simulink model "ROPOD_dynamic_model_sim_Wheel_Input"  (R2016b)
settings: Solver=FixedStepAuto  StartTime=0.0  StopTime=timesim(end)  FixedStep=Ts  MaxStep=1e-3  RelTol=1e-3
values from neighbouring files (symbols this model uses):
  ropod_dynmodel_pv = struct2array(ropod_dynmodel_param)    [set_ropod_configparams_sim.m]
(part 4 of 4)

== matlab function ROPOD_dynamic_model_sim_Wheel_Input/Feedback Linearization/m_vector_c ==
  data: ropod_dynmodel_pv input; m output; qin input; dqin input
function m   = m_vector( ropod_dynmodel_pv, qin, dqin)
%ROPOD_JACOBIAN Summary of this function goes here
%   Detailed explanation goes here


r_w     = ropod_dynmodel_pv(1);
s_w     = ropod_dynmodel_pv(2);
d_w     = ropod_dynmodel_pv(3);
l_CW    = ropod_dynmodel_pv(4);

Mr = ropod_dynmodel_pv(5);
Ir = ropod_dynmodel_pv(6);
Mwma = ropod_dynmodel_pv(7);
Iwma = ropod_dynmodel_pv(8);
Mwca = ropod_dynmodel_pv(9);
Iwca = ropod_dynmodel_pv(10);
Mw   = ropod_dynmodel_pv(11);
Iwz  = ropod_dynmodel_pv(12);
Iwp  = ropod_dynmodel_pv(13);

% Map state vector to the corresponfing variables
xc      = qin(1);
yc      = qin(2);
theta   = qin(3);
delta   = qin(4:7);
varphi  = qin(8:15);

% Map state vector to the corresponfing variables
dxc      = dqin(1);
dyc      = dqin(2);
dtheta   = dqin(3);
ddelta   = dqin(4:7);
dvarphi  = dqin(8:15);

delta1 = delta(1);
delta2 = delta(2);
delta3 = delta(3);
delta4 = delta(4);

ddelta1 = ddelta(1);
ddelta2 = ddelta(2);
ddelta3 = ddelta(3);
ddelta4 = ddelta(4);

m = [
                                                                                                                                                                                                                                                                                                                                                                                                                                                                                                                                                                                                                                                                                                                                                                                                                                                                                                                                                                                                                                                                                                                                                                                                                                                                                                                                                                                                                                                                                                                                                                                                                                                                                                                                                                                                                                                                                                                                                                                                                                                                                                                                                                                                                                                                                                                                                                                                                                                                                                                                                                                                                                      dyc*((Iwp*(cos(delta1 + theta) - (d_w*sin(delta1 + theta))/(2*s_w))*(cos(delta1 + theta)*(ddelta1 + dtheta) - (d_w*sin(delta1 + theta)*(ddelta1 + dtheta))/(2*s_w)))/r_w^2 + (Iwp*(cos(delta1 + theta) + (d_w*sin(delta1 + theta))/(2*s_w))*(cos(delta1 + theta)*(ddelta1 + dtheta) + (d_w*sin(delta1 + theta)*(ddelta1 + dtheta))/(2*s_w)))/r_w^2 + (Iwp*(cos(delta2 + theta) - (d_w*sin(delta2 + theta))/(2*s_w))*(cos(delta2 + theta)*(ddelta2 + dtheta) - (d_w*sin(delta2 + theta)*(ddelta2 + dtheta))/(2*s_w)))/r_w^2 + (Iwp*(cos(delta2 + theta) + (d_w*sin(delta2 + theta))/(2*s_w))*(cos(delta2 + theta)*(ddelta2 + dtheta) + (d_w*sin(delta2 + theta)*(ddelta2 + dtheta))/(2*s_w)))/r_w^2 + (Iwp*(cos(delta3 + theta) - (d_w*sin(delta3 + theta))/(2*s_w))*(cos(delta3 + theta)*(ddelta3 + dtheta) - (d_w*sin(delta3 + theta)*(ddelta3 + dtheta))/(2*s_w)))/r_w^2 + (Iwp*(cos(delta3 + theta) + (d_w*sin(delta3 + theta))/(2*s_w))*(cos(delta3 + theta)*(ddelta3 + dtheta) + (d_w*sin(delta3 + theta)*(ddelta3 + dtheta))/(2*s_w)))/r_w^2 + (Iwp*(cos(delta4 + theta) - (d_w*sin(delta4 + theta))/(2*s_w))*(cos(delta4 + theta)*(ddelta4 + dtheta) - (d_w*sin(delta4 + theta)*(ddelta4 + dtheta))/(2*s_w)))/r_w^2 + (Iwp*(cos(delta4 + theta) + (d_w*sin(delta4 + theta))/(2*s_w))*(cos(delta4 + theta)*(ddelta4 + dtheta) + (d_w*sin(delta4 + theta)*(ddelta4 + dtheta))/(2*s_w)))/r_w^2 - (sin(delta1 + theta)*(ddelta1 + dtheta)*(2*Mw*s_w*cos(delta1)*sin(theta) - (sin(delta1 + theta)*(Iwca + Iwma + 2*Iwz + (Mw*d_w^2)/2 + 2*Mw*s_w^2 + (Mwca*s_w^2)/4 + Mwma*s_w^2))/s_w + 2*Mw*s_w*sin(delta1)*cos(theta) + (Mwca*s_w*cos(delta1)*sin(theta))/2 + (Mwca*s_w*sin(delta1)*cos(theta))/2 + Mwma*s_w*cos(delta1)*sin(theta) + Mwma*s_w*sin(delta1)*cos(theta)))/s_w - (sin(delta2 + theta)*(ddelta2 + dtheta)*(2*Mw*s_w*cos(delta2)*sin(theta) - (sin(delta2 + theta)*(Iwca + Iwma + 2*Iwz + (Mw*d_w^2)/2 + 2*Mw*s_w^2 + (Mwca*s_w^2)/4 + Mwma*s_w^2))/s_w + 2*Mw*s_w*sin(delta2)*cos(theta) + (Mwca*s_w*cos(delta2)*sin(theta))/2 + (Mwca*s_w*sin(delta2)*cos(theta))/2 + Mwma*s_w*cos(delta2)*sin(theta) + Mwma*s_w*sin(delta2)*cos(theta)))/s_w - (sin(delta3 + theta)*(ddelta3 + dtheta)*(2*Mw*s_w*cos(delta3)*sin(theta) - (sin(delta3 + theta)*(Iwca + Iwma + 2*Iwz + (Mw*d_w^2)/2 + 2*Mw*s_w^2 + (Mwca*s_w^2)/4 + Mwma*s_w^2))/s_w + 2*Mw*s_w*sin(delta3)*cos(theta) + (Mwca*s_w*cos(delta3)*sin(theta))/2 + (Mwca*s_w*sin(delta3)*cos(theta))/2 + Mwma*s_w*cos(delta3)*sin(theta) + Mwma*s_w*sin(delta3)*cos(theta)))/s_w - (sin(delta4 + theta)*(ddelta4 + dtheta)*(2*Mw*s_w*cos(delta4)*sin(theta) - (sin(delta4 + theta)*(Iwca + Iwma + 2*Iwz + (Mw*d_w^2)/2 + 2*Mw*s_w^2 + (Mwca*s_w^2)/4 + Mwma*s_w^2))/s_w + 2*Mw*s_w*sin(delta4)*cos(theta) + (Mwca*s_w*cos(delta4)*sin(theta))/2 + (Mwca*s_w*sin(delta4)*cos(theta))/2 + Mwma*s_w*cos(delta4)*sin(theta) + Mwma*s_w*sin(delta4)*cos(theta)))/s_w) - dtheta*(((ddelta1*l_CW*sin(delta1) - ddelta1*l_CW*cos(delta1))*(2*Mw*s_w*cos(delta1)*sin(theta) - (sin(delta1 + theta)*(Iwca + Iwma + 2*Iwz + (Mw*d_w^2)/2 + 2*Mw*s_w^2 + (Mwca*s_w^2)/4 + Mwma*s_w^2))/s_w + 2*Mw*s_w*sin(delta1)*cos(theta) + (Mwca*s_w*cos(delta1)*sin(theta))/2 + (Mwca*s_w*sin(delta1)*cos(theta))/2 + Mwma*s_w*cos(delta1)*sin(theta) + Mwma*s_w*sin(delta1)*cos(theta)))/s_w + ((ddelta2*l_CW*sin(delta2) + ddelta2*l_CW*cos(delta2))*(2*Mw*s_w*cos(delta2)*sin(theta) - (sin(delta2 + theta)*(Iwca + Iwma + 2*Iwz + (Mw*d_w^2)/2 + 2*Mw*s_w^2 + (Mwca*s_w^2)/4 + Mwma*s_w^2))/s_w + 2*Mw*s_w*sin(delta2)*cos(theta) + (Mwca*s_w*cos(delta2)*sin(theta))/2 + (Mwca*s_w*sin(delta2)*cos(theta))/2 + Mwma*s_w*cos(delta2)*sin(theta) + Mwma*s_w*sin(delta2)*cos(theta)))/s_w - ((ddelta3*l_CW*sin(delta3) - ddelta3*l_CW*cos(delta3))*(2*Mw*s_w*cos(delta3)*sin(theta) - (sin(delta3 + theta)*(Iwca + Iwma + 2*Iwz + (Mw*d_w^2)/2 + 2*Mw*s_w^2 + (Mwca*s_w^2)/4 + Mwma*s_w^2))/s_w + 2*Mw*s_w*sin(delta3)*cos(theta) + (Mwca*s_w*cos(delta3)*sin(theta))/2 + (Mwca*s_w*sin(delta3)*cos(theta))/2 + Mwma*s_w*cos(delta3)*sin(theta) + Mwma*s_w*sin(delta3)*cos(theta)))/s_w - ((ddelta4*l_CW*sin(delta4) + ddelta4*l_CW*cos(delta4))*(2*Mw*s_w*cos(delta4)*sin(theta) - (sin(delta4 + theta)*(Iwca + Iwma + 2*Iwz + (Mw*d_w^2)/2 + 2*Mw*s_w^2 + (Mwca*s_w^2)/4 + Mwma*s_w^2))/s_w + 2*Mw*s_w*sin(delta4)*cos(theta) + (Mwca*s_w*cos(delta4)*sin(theta))/2 + (Mwca*s_w*sin(delta4)*cos(theta))/2 + Mwma*s_w*cos(delta4)*sin(theta) + Mwma*s_w*sin(delta4)*cos(theta)))/s_w - (Iwp*l_CW*(cos(delta1 + theta) - (d_w*sin(delta1 + theta))/(2*s_w))*(2*ddelta1*s_w*sin(delta1) - d_w*ddelta1*sin(delta1) + d_w*ddelta1*cos(delta1) + 2*ddelta1*s_w*cos(delta1)))/(2*r_w^2*s_w) - (Iwp*l_CW*(cos(delta1 + theta) + (d_w*sin(delta1 + theta))/(2*s_w))*(d_w*ddelta1*sin(delta1) + 2*ddelta1*s_w*sin(delta1) - d_w*ddelta1*cos(delta1) + 2*ddelta1*s_w*cos(delta1)))/(2*r_w^2*s_w) + (Iwp*l_CW*(cos(delta2 + theta) - (d_w*sin(delta2 + theta))/(2*s_w))*(d_w*ddelta2*sin(delta2) + 2*ddelta2*s_w*sin(delta2) + d_w*ddelta2*cos(delta2) - 2*ddelta2*s_w*cos(delta2)))/(2*r_w^2*s_w) - (Iwp*l_CW*(cos(delta2 + theta) + (d_w*sin(delta2 + theta))/(2*s_w))*(d_w*ddelta2*sin(delta2) - 2*ddelta2*s_w*sin(delta2) + d_w*ddelta2*cos(delta2) + 2*ddelta2*s_w*cos(delta2)))/(2*r_w^2*s_w) + (Iwp*l_CW*(cos(delta3 + theta) - (d_w*sin(delta3 + theta))/(2*s_w))*(2*ddelta3*s_w*sin(delta3) - d_w*ddelta3*sin(delta3) + d_w*ddelta3*cos(delta3) + 2*ddelta3*s_w*cos(delta3)))/(2*r_w^2*s_w) + (Iwp*l_CW*(cos(delta3 + theta) + (d_w*sin(delta3 + theta))/(2*s_w))*(d_w*ddelta3*sin(delta3) + 2*ddelta3*s_w*sin(delta3) - d_w*ddelta3*cos(delta3) + 2*ddelta3*s_w*cos(delta3)))/(2*r_w^2*s_w) - (Iwp*l_CW*(cos(delta4 + theta) - (d_w*sin(delta4 + theta))/(2*s_w))*(d_w*ddelta4*sin(delta4) + 2*ddelta4*s_w*sin(delta4) + d_w*ddelta4*cos(delta4) - 2*ddelta4*s_w*cos(delta4)))/(2*r_w^2*s_w) + (Iwp*l_CW*(cos(delta4 + theta) + (d_w*sin(delta4 + theta))/(2*s_w))*(d_w*ddelta4*sin(delta4) - 2*ddelta4*s_w*sin(delta4) + d_w*ddelta4*cos(delta4) + 2*ddelta4*s_w*cos(delta4)))/(2*r_w^2*s_w)) - dxc*((cos(delta1 + theta)*(ddelta1 + dtheta)*(2*Mw*s_w*cos(delta1)*sin(theta) - (sin(delta1 + theta)*(Iwca + Iwma + 2*Iwz + (Mw*d_w^2)/2 + 2*Mw*s_w^2 + (Mwca*s_w^2)/4 + Mwma*s_w^2))/s_w + 2*Mw*s_w*sin(delta1)*cos(theta) + (Mwca*s_w*cos(delta1)*sin(theta))/2 + (Mwca*s_w*sin(delta1)*cos(theta))/2 + Mwma*s_w*cos(delta1)*sin(theta) + Mwma*s_w*sin(delta1)*cos(theta)))/s_w + (cos(delta2 + theta)*(ddelta2 + dtheta)*(2*Mw*s_w*cos(delta2)*sin(theta) - (sin(delta2 + theta)*(Iwca + Iwma + 2*Iwz + (Mw*d_w^2)/2 + 2*Mw*s_w^2 + (Mwca*s_w^2)/4 + Mwma*s_w^2))/s_w + 2*Mw*s_w*sin(delta2)*cos(theta) + (Mwca*s_w*cos(delta2)*sin(theta))/2 + (Mwca*s_w*sin(delta2)*cos(theta))/2 + Mwma*s_w*cos(delta2)*sin(theta) + Mwma*s_w*sin(delta2)*cos(theta)))/s_w + (cos(delta3 + theta)*(ddelta3 + dtheta)*(2*Mw*s_w*cos(delta3)*sin(theta) - (sin(delta3 + theta)*(Iwca + Iwma + 2*Iwz + (Mw*d_w^2)/2 + 2*Mw*s_w^2 + (Mwca*s_w^2)/4 + Mwma*s_w^2))/s_w + 2*Mw*s_w*sin(delta3)*cos(theta) + (Mwca*s_w*cos(delta3)*sin(theta))/2 + (Mwca*s_w*sin(delta3)*cos(theta))/2 + Mwma*s_w*cos(delta3)*sin(theta) + Mwma*s_w*sin(delta3)*cos(theta)))/s_w + (cos(delta4 + theta)*(ddelta4 + dtheta)*(2*Mw*s_w*cos(delta4)*sin(theta) - (sin(delta4 + theta)*(Iwca + Iwma + 2*Iwz + (Mw*d_w^2)/2 + 2*Mw*s_w^2 + (Mwca*s_w^2)/4 + Mwma*s_w^2))/s_w + 2*Mw*s_w*sin(delta4)*cos(theta) + (Mwca*s_w*cos(delta4)*sin(theta))/2 + (Mwca*s_w*sin(delta4)*cos(theta))/2 + Mwma*s_w*cos(delta4)*sin(theta) + Mwma*s_w*sin(delta4)*cos(theta)))/s_w + (Iwp*(cos(delta1 + theta) - (d_w*sin(delta1 + theta))/(2*s_w))*(sin(delta1 + theta)*(ddelta1 + dtheta) + (d_w*cos(delta1 + theta)*(ddelta1 + dtheta))/(2*s_w)))/r_w^2 + (Iwp*(cos(delta1 + theta) + (d_w*sin(delta1 + theta))/(2*s_w))*(sin(delta1 + theta)*(ddelta1 + dtheta) - (d_w*cos(delta1 + theta)*(ddelta1 + dtheta))/(2*s_w)))/r_w^2 + (Iwp*(cos(delta2 + theta) - (d_w*sin(delta2 + theta))/(2*s_w))*(sin(delta2 + theta)*(ddelta2 + dtheta) + (d_w*cos(delta2 + theta)*(ddelta2 + dtheta))/(2*s_w)))/r_w^2 + (Iwp*(cos(delta2 + theta) + (d_w*sin(delta2 + theta))/(2*s_w))*(sin(delta2 + theta)*(ddelta2 + dtheta) - (d_w*cos(delta2 + theta)*(ddelta2 + dtheta))/(2*s_w)))/r_w^2 + (Iwp*(cos(delta3 + theta) - (d_w*sin(delta3 + theta))/(2*s_w))*(sin(delta3 + theta)*(ddelta3 + dtheta) + (d_w*cos(delta3 + theta)*(ddelta3 + dtheta))/(2*s_w)))/r_w^2 + (Iwp*(cos(delta3 + theta) + (d_w*sin(delta3 + theta))/(2*s_w))*(sin(delta3 + theta)*(ddelta3 + dtheta) - (d_w*cos(delta3 + theta)*(ddelta3 + dtheta))/(2*s_w)))/r_w^2 + (Iwp*(cos(delta4 + theta) - (d_w*sin(delta4 + theta))/(2*s_w))*(sin(delta4 + theta)*(ddelta4 + dtheta) + (d_w*cos(delta4 + theta)*(ddelta4 + dtheta))/(2*s_w)))/r_w^2 + (Iwp*(cos(delta4 + theta) + (d_w*sin(delta4 + theta))/(2*s_w))*(sin(delta4 + theta)*(ddelta4 + dtheta) - (d_w*cos(delta4 + theta)*(ddelta4 + dtheta))/(2*s_w)))/r_w^2) + (s_w*(4*Mw + Mwca + 2*Mwma)*(cos(delta1 + theta)*(dtheta*((l_CW*cos(delta1) + l_CW*sin(delta1))/s_w - 1) + (dyc*cos(delta1 + theta))/s_w - (dxc*sin(delta1 + theta))/s_w)^2 + cos(delta2 + theta)*(dtheta*((l_CW*cos(delta2) - l_CW*sin(delta2))/s_w - 1) + (dyc*cos(delta2 + theta))/s_w - (dxc*sin(delta2 + theta))/s_w)^2 + cos(delta3 + theta)*(dtheta*((l_CW*cos(delta3) + l_CW*sin(delta3))/s_w + 1) - (dyc*cos(delta3 + theta))/s_w + (dxc*sin(delta3 + theta))/s_w)^2 + cos(delta4 + theta)*(dtheta*((l_CW*cos(delta4) - l_CW*sin(delta4))/s_w + 1) - (dyc*cos(delta4 + theta))/s_w + (dxc*sin(delta4 + theta))/s_w)^2 + dtheta^2*cos(delta1 + theta) + dtheta^2*cos(delta2 + theta) + dtheta^2*cos(delta3 + theta) + dtheta^2*cos(delta4 + theta) + 2*dtheta*cos(delta1 + theta)*(dtheta*((l_CW*cos(delta1) + l_CW*sin(delta1))/s_w - 1) + (dyc*cos(delta1 + theta))/s_w - (dxc*sin(delta1 + theta))/s_w) + 2*dtheta*cos(delta2 + theta)*(dtheta*((l_CW*cos(delta2) - l_CW*sin(delta2))/s_w - 1) + (dyc*cos(delta2 + theta))/s_w - (dxc*sin(delta2 + theta))/s_w) - 2*dtheta*cos(delta3 + theta)*(dtheta*((l_CW*cos(delta3) + l_CW*sin(delta3))/s_w + 1) - (dyc*cos(delta3 + theta))/s_w + (dxc*sin(delta3 + theta))/s_w) - 2*dtheta*cos(delta4 + theta)*(dtheta*((l_CW*cos(delta4) - l_CW*sin(delta4))/s_w + 1) - (dyc*cos(delta4 + theta))/s_w + (dxc*sin(delta4 + theta))/s_w)))/2 - (2^(1/2)*dtheta^2*l_CW*sin(delta1 + theta)*cos(delta1 + pi/4)*(4*Mw + Mwca + 2*Mwma))/2 + (2^(1/2)*dtheta^2*l_CW*sin(delta3 + theta)*cos(delta3 + pi/4)*(4*Mw + Mwca + 2*Mwma))/2 + (2^(1/2)*dtheta^2*l_CW*sin(delta2 + theta)*sin(delta2 + pi/4)*(4*Mw + Mwca + 2*Mwma))/2 - (2^(1/2)*dtheta^2*l_CW*sin(delta4 + theta)*sin(delta4 + pi/4)*(4*Mw + Mwca + 2*Mwma))/2 ;
                                                                                                                                                                                                                                                                                                                                                                                                                                                                                                                                                                                                                                                                                                                                                                                                                                                                                                                                                                                                                                                                                                                                                                                                                                                                                                                                                                                                                                                                                                                                                                                                                                                                                                                                                                                                                                                                                                                                                                                                                                                                                                                                                                                                                                                                                                                                                                                                                                                                                                                                                                                                                                      dyc*((Iwp*(sin(delta1 + theta) - (d_w*cos(delta1 + theta))/(2*s_w))*(cos(delta1 + theta)*(ddelta1 + dtheta) + (d_w*sin(delta1 + theta)*(ddelta1 + dtheta))/(2*s_w)))/r_w^2 - (sin(delta2 + theta)*(ddelta2 + dtheta)*((cos(delta2 + theta)*(Iwca + Iwma + 2*Iwz + (Mw*d_w^2)/2 + 2*Mw*s_w^2 + (Mwca*s_w^2)/4 + Mwma*s_w^2))/s_w - 2*Mw*s_w*cos(delta2)*cos(theta) - (Mwca*s_w*cos(delta2)*cos(theta))/2 - Mwma*s_w*cos(delta2)*cos(theta) + 2*Mw*s_w*sin(delta2)*sin(theta) + (Mwca*s_w*sin(delta2)*sin(theta))/2 + Mwma*s_w*sin(delta2)*sin(theta)))/s_w - (sin(delta3 + theta)*(ddelta3 + dtheta)*((cos(delta3 + theta)*(Iwca + Iwma + 2*Iwz + (Mw*d_w^2)/2 + 2*Mw*s_w^2 + (Mwca*s_w^2)/4 + Mwma*s_w^2))/s_w - 2*Mw*s_w*cos(delta3)*cos(theta) - (Mwca*s_w*cos(delta3)*cos(theta))/2 - Mwma*s_w*cos(delta3)*cos(theta) + 2*Mw*s_w*sin(delta3)*sin(theta) + (Mwca*s_w*sin(delta3)*sin(theta))/2 + Mwma*s_w*sin(delta3)*sin(theta)))/s_w - (sin(delta4 + theta)*(ddelta4 + dtheta)*((cos(delta4 + theta)*(Iwca + Iwma + 2*Iwz + (Mw*d_w^2)/2 + 2*Mw*s_w^2 + (Mwca*s_w^2)/4 + Mwma*s_w^2))/s_w - 2*Mw*s_w*cos(delta4)*cos(theta) - (Mwca*s_w*cos(delta4)*cos(theta))/2 - Mwma*s_w*cos(delta4)*cos(theta) + 2*Mw*s_w*sin(delta4)*sin(theta) + (Mwca*s_w*sin(delta4)*sin(theta))/2 + Mwma*s_w*sin(delta4)*sin(theta)))/s_w - (sin(delta1 + theta)*(ddelta1 + dtheta)*((cos(delta1 + theta)*(Iwca + Iwma + 2*Iwz + (Mw*d_w^2)/2 + 2*Mw*s_w^2 + (Mwca*s_w^2)/4 + Mwma*s_w^2))/s_w - 2*Mw*s_w*cos(delta1)*cos(theta) - (Mwca*s_w*cos(delta1)*cos(theta))/2 - Mwma*s_w*cos(delta1)*cos(theta) + 2*Mw*s_w*sin(delta1)*sin(theta) + (Mwca*s_w*sin(delta1)*sin(theta))/2 + Mwma*s_w*sin(delta1)*sin(theta)))/s_w + (Iwp*(sin(delta1 + theta) + (d_w*cos(delta1 + theta))/(2*s_w))*(cos(delta1 + theta)*(ddelta1 + dtheta) - (d_w*sin(delta1 + theta)*(ddelta1 + dtheta))/(2*s_w)))/r_w^2 + (Iwp*(sin(delta2 + theta) - (d_w*cos(delta2 + theta))/(2*s_w))*(cos(delta2 + theta)*(ddelta2 + dtheta) + (d_w*sin(delta2 + theta)*(ddelta2 + dtheta))/(2*s_w)))/r_w^2 + (Iwp*(sin(delta2 + theta) + (d_w*cos(delta2 + theta))/(2*s_w))*(cos(delta2 + theta)*(ddelta2 + dtheta) - (d_w*sin(delta2 + theta)*(ddelta2 + dtheta))/(2*s_w)))/r_w^2 + (Iwp*(sin(delta3 + theta) - (d_w*cos(delta3 + theta))/(2*s_w))*(cos(delta3 + theta)*(ddelta3 + dtheta) + (d_w*sin(delta3 + theta)*(ddelta3 + dtheta))/(2*s_w)))/r_w^2 + (Iwp*(sin(delta3 + theta) + (d_w*cos(delta3 + theta))/(2*s_w))*(cos(delta3 + theta)*(ddelta3 + dtheta) - (d_w*sin(delta3 + theta)*(ddelta3 + dtheta))/(2*s_w)))/r_w^2 + (Iwp*(sin(delta4 + theta) - (d_w*cos(delta4 + theta))/(2*s_w))*(cos(delta4 + theta)*(ddelta4 + dtheta) + (d_w*sin(delta4 + theta)*(ddelta4 + dtheta))/(2*s_w)))/r_w^2 + (Iwp*(sin(delta4 + theta) + (d_w*cos(delta4 + theta))/(2*s_w))*(cos(delta4 + theta)*(ddelta4 + dtheta) - (d_w*sin(delta4 + theta)*(ddelta4 + dtheta))/(2*s_w)))/r_w^2) - dxc*((cos(delta1 + theta)*(ddelta1 + dtheta)*((cos(delta1 + theta)*(Iwca + Iwma + 2*Iwz + (Mw*d_w^2)/2 + 2*Mw*s_w^2 + (Mwca*s_w^2)/4 + Mwma*s_w^2))/s_w - 2*Mw*s_w*cos(delta1)*cos(theta) - (Mwca*s_w*cos(delta1)*cos(theta))/2 - Mwma*s_w*cos(delta1)*cos(theta) + 2*Mw*s_w*sin(delta1)*sin(theta) + (Mwca*s_w*sin(delta1)*sin(theta))/2 + Mwma*s_w*sin(delta1)*sin(theta)))/s_w + (cos(delta2 + theta)*(ddelta2 + dtheta)*((cos(delta2 + theta)*(Iwca + Iwma + 2*Iwz + (Mw*d_w^2)/2 + 2*Mw*s_w^2 + (Mwca*s_w^2)/4 + Mwma*s_w^2))/s_w - 2*Mw*s_w*cos(delta2)*cos(theta) - (Mwca*s_w*cos(delta2)*cos(theta))/2 - Mwma*s_w*cos(delta2)*cos(theta) + 2*Mw*s_w*sin(delta2)*sin(theta) + (Mwca*s_w*sin(delta2)*sin(theta))/2 + Mwma*s_w*sin(delta2)*sin(theta)))/s_w + (cos(delta3 + theta)*(ddelta3 + dtheta)*((cos(delta3 + theta)*(Iwca + Iwma + 2*Iwz + (Mw*d_w^2)/2 + 2*Mw*s_w^2 + (Mwca*s_w^2)/4 + Mwma*s_w^2))/s_w - 2*Mw*s_w*cos(delta3)*cos(theta) - (Mwca*s_w*cos(delta3)*cos(theta))/2 - Mwma*s_w*cos(delta3)*cos(theta) + 2*Mw*s_w*sin(delta3)*sin(theta) + (Mwca*s_w*sin(delta3)*sin(theta))/2 + Mwma*s_w*sin(delta3)*sin(theta)))/s_w + (cos(delta4 + theta)*(ddelta4 + dtheta)*((cos(delta4 + theta)*(Iwca + Iwma + 2*Iwz + (Mw*d_w^2)/2 + 2*Mw*s_w^2 + (Mwca*s_w^2)/4 + Mwma*s_w^2))/s_w - 2*Mw*s_w*cos(delta4)*cos(theta) - (Mwca*s_w*cos(delta4)*cos(theta))/2 - Mwma*s_w*cos(delta4)*cos(theta) + 2*Mw*s_w*sin(delta4)*sin(theta) + (Mwca*s_w*sin(delta4)*sin(theta))/2 + Mwma*s_w*sin(delta4)*sin(theta)))/s_w + (Iwp*(sin(delta1 + theta) - (d_w*cos(delta1 + theta))/(2*s_w))*(sin(delta1 + theta)*(ddelta1 + dtheta) - (d_w*cos(delta1 + theta)*(ddelta1 + dtheta))/(2*s_w)))/r_w^2 + (Iwp*(sin(delta1 + theta) + (d_w*cos(delta1 + theta))/(2*s_w))*(sin(delta1 + theta)*(ddelta1 + dtheta) + (d_w*cos(delta1 + theta)*(ddelta1 + dtheta))/(2*s_w)))/r_w^2 + (Iwp*(sin(delta2 + theta) - (d_w*cos(delta2 + theta))/(2*s_w))*(sin(delta2 + theta)*(ddelta2 + dtheta) - (d_w*cos(delta2 + theta)*(ddelta2 + dtheta))/(2*s_w)))/r_w^2 + (Iwp*(sin(delta2 + theta) + (d_w*cos(delta2 + theta))/(2*s_w))*(sin(delta2 + theta)*(ddelta2 + dtheta) + (d_w*cos(delta2 + theta)*(ddelta2 + dtheta))/(2*s_w)))/r_w^2 + (Iwp*(sin(delta3 + theta) - (d_w*cos(delta3 + theta))/(2*s_w))*(sin(delta3 + theta)*(ddelta3 + dtheta) - (d_w*cos(delta3 + theta)*(ddelta3 + dtheta))/(2*s_w)))/r_w^2 + (Iwp*(sin(delta3 + theta) + (d_w*cos(delta3 + theta))/(2*s_w))*(sin(delta3 + theta)*(ddelta3 + dtheta) + (d_w*cos(delta3 + theta)*(ddelta3 + dtheta))/(2*s_w)))/r_w^2 + (Iwp*(sin(delta4 + theta) - (d_w*cos(delta4 + theta))/(2*s_w))*(sin(delta4 + theta)*(ddelta4 + dtheta) - (d_w*cos(delta4 + theta)*(ddelta4 + dtheta))/(2*s_w)))/r_w^2 + (Iwp*(sin(delta4 + theta) + (d_w*cos(delta4 + theta))/(2*s_w))*(sin(delta4 + theta)*(ddelta4 + dtheta) + (d_w*cos(delta4 + theta)*(ddelta4 + dtheta))/(2*s_w)))/r_w^2) - dtheta*(((ddelta1*l_CW*sin(delta1) - ddelta1*l_CW*cos(delta1))*((cos(delta1 + theta)*(Iwca + Iwma + 2*Iwz + (Mw*d_w^2)/2 + 2*Mw*s_w^2 + (Mwca*s_w^2)/4 + Mwma*s_w^2))/s_w - 2*Mw*s_w*cos(delta1)*cos(theta) - (Mwca*s_w*cos(delta1)*cos(theta))/2 - Mwma*s_w*cos(delta1)*cos(theta) + 2*Mw*s_w*sin(delta1)*sin(theta) + (Mwca*s_w*sin(delta1)*sin(theta))/2 + Mwma*s_w*sin(delta1)*sin(theta)))/s_w + ((ddelta2*l_CW*sin(delta2) + ddelta2*l_CW*cos(delta2))*((cos(delta2 + theta)*(Iwca + Iwma + 2*Iwz + (Mw*d_w^2)/2 + 2*Mw*s_w^2 + (Mwca*s_w^2)/4 + Mwma*s_w^2))/s_w - 2*Mw*s_w*cos(delta2)*cos(theta) - (Mwca*s_w*cos(delta2)*cos(theta))/2 - Mwma*s_w*cos(delta2)*cos(theta) + 2*Mw*s_w*sin(delta2)*sin(theta) + (Mwca*s_w*sin(delta2)*sin(theta))/2 + Mwma*s_w*sin(delta2)*sin(theta)))/s_w - ((ddelta3*l_CW*sin(delta3) - ddelta3*l_CW*cos(delta3))*((cos(delta3 + theta)*(Iwca + Iwma + 2*Iwz + (Mw*d_w^2)/2 + 2*Mw*s_w^2 + (Mwca*s_w^2)/4 + Mwma*s_w^2))/s_w - 2*Mw*s_w*cos(delta3)*cos(theta) - (Mwca*s_w*cos(delta3)*cos(theta))/2 - Mwma*s_w*cos(delta3)*cos(theta) + 2*Mw*s_w*sin(delta3)*sin(theta) + (Mwca*s_w*sin(delta3)*sin(theta))/2 + Mwma*s_w*sin(delta3)*sin(theta)))/s_w - ((ddelta4*l_CW*sin(delta4) + ddelta4*l_CW*cos(delta4))*((cos(delta4 + theta)*(Iwca + Iwma + 2*Iwz + (Mw*d_w^2)/2 + 2*Mw*s_w^2 + (Mwca*s_w^2)/4 + Mwma*s_w^2))/s_w - 2*Mw*s_w*cos(delta4)*cos(theta) - (Mwca*s_w*cos(delta4)*cos(theta))/2 - Mwma*s_w*cos(delta4)*cos(theta) + 2*Mw*s_w*sin(delta4)*sin(theta) + (Mwca*s_w*sin(delta4)*sin(theta))/2 + Mwma*s_w*sin(delta4)*sin(theta)))/s_w - (Iwp*l_CW*(sin(delta1 + theta) - (d_w*cos(delta1 + theta))/(2*s_w))*(d_w*ddelta1*sin(delta1) + 2*ddelta1*s_w*sin(delta1) - d_w*ddelta1*cos(delta1) + 2*ddelta1*s_w*cos(delta1)))/(2*r_w^2*s_w) - (Iwp*l_CW*(sin(delta1 + theta) + (d_w*cos(delta1 + theta))/(2*s_w))*(2*ddelta1*s_w*sin(delta1) - d_w*ddelta1*sin(delta1) + d_w*ddelta1*cos(delta1) + 2*ddelta1*s_w*cos(delta1)))/(2*r_w^2*s_w) - (Iwp*l_CW*(sin(delta2 + theta) - (d_w*cos(delta2 + theta))/(2*s_w))*(d_w*ddelta2*sin(delta2) - 2*ddelta2*s_w*sin(delta2) + d_w*ddelta2*cos(delta2) + 2*ddelta2*s_w*cos(delta2)))/(2*r_w^2*s_w) + (Iwp*l_CW*(sin(delta2 + theta) + (d_w*cos(delta2 + theta))/(2*s_w))*(d_w*ddelta2*sin(delta2) + 2*ddelta2*s_w*sin(delta2) + d_w*ddelta2*cos(delta2) - 2*ddelta2*s_w*cos(delta2)))/(2*r_w^2*s_w) + (Iwp*l_CW*(sin(delta3 + theta) - (d_w*cos(delta3 + theta))/(2*s_w))*(d_w*ddelta3*sin(delta3) + 2*ddelta3*s_w*sin(delta3) - d_w*ddelta3*cos(delta3) + 2*ddelta3*s_w*cos(delta3)))/(2*r_w^2*s_w) + (Iwp*l_CW*(sin(delta3 + theta) + (d_w*cos(delta3 + theta))/(2*s_w))*(2*ddelta3*s_w*sin(delta3) - d_w*ddelta3*sin(delta3) + d_w*ddelta3*cos(delta3) + 2*ddelta3*s_w*cos(delta3)))/(2*r_w^2*s_w) + (Iwp*l_CW*(sin(delta4 + theta) - (d_w*cos(delta4 + theta))/(2*s_w))*(d_w*ddelta4*sin(delta4) - 2*ddelta4*s_w*sin(delta4) + d_w*ddelta4*cos(delta4) + 2*ddelta4*s_w*cos(delta4)))/(2*r_w^2*s_w) - (Iwp*l_CW*(sin(delta4 + theta) + (d_w*cos(delta4 + theta))/(2*s_w))*(d_w*ddelta4*sin(delta4) + 2*ddelta4*s_w*sin(delta4) + d_w*ddelta4*cos(delta4) - 2*ddelta4*s_w*cos(delta4)))/(2*r_w^2*s_w)) + (s_w*(4*Mw + Mwca + 2*Mwma)*(sin(delta1 + theta)*(dtheta*((l_CW*cos(delta1) + l_CW*sin(delta1))/s_w - 1) + (dyc*cos(delta1 + theta))/s_w - (dxc*sin(delta1 + theta))/s_w)^2 + sin(delta2 + theta)*(dtheta*((l_CW*cos(delta2) - l_CW*sin(delta2))/s_w - 1) + (dyc*cos(delta2 + theta))/s_w - (dxc*sin(delta2 + theta))/s_w)^2 + sin(delta3 + theta)*(dtheta*((l_CW*cos(delta3) + l_CW*sin(delta3))/s_w + 1) - (dyc*cos(delta3 + theta))/s_w + (dxc*sin(delta3 + theta))/s_w)^2 + sin(delta4 + theta)*(dtheta*((l_CW*cos(delta4) - l_CW*sin(delta4))/s_w + 1) - (dyc*cos(delta4 + theta))/s_w + (dxc*sin(delta4 + theta))/s_w)^2 + dtheta^2*sin(delta1 + theta) + dtheta^2*sin(delta2 + theta) + dtheta^2*sin(delta3 + theta) + dtheta^2*sin(delta4 + theta) + 2*dtheta*sin(delta1 + theta)*(dtheta*((l_CW*cos(delta1) + l_CW*sin(delta1))/s_w - 1) + (dyc*cos(delta1 + theta))/s_w - (dxc*sin(delta1 + theta))/s_w) + 2*dtheta*sin(delta2 + theta)*(dtheta*((l_CW*cos(delta2) - l_CW*sin(delta2))/s_w - 1) + (dyc*cos(delta2 + theta))/s_w - (dxc*sin(delta2 + theta))/s_w) - 2*dtheta*sin(delta3 + theta)*(dtheta*((l_CW*cos(delta3) + l_CW*sin(delta3))/s_w + 1) - (dyc*cos(delta3 + theta))/s_w + (dxc*sin(delta3 + theta))/s_w) - 2*dtheta*sin(delta4 + theta)*(dtheta*((l_CW*cos(delta4) - l_CW*sin(delta4))/s_w + 1) - (dyc*cos(delta4 + theta))/s_w + (dxc*sin(delta4 + theta))/s_w)))/2 + (2^(1/2)*dtheta^2*l_CW*cos(delta1 + theta)*cos(delta1 + pi/4)*(4*Mw + Mwca + 2*Mwma))/2 - (2^(1/2)*dtheta^2*l_CW*cos(delta3 + theta)*cos(delta3 + pi/4)*(4*Mw + Mwca + 2*Mwma))/2 - (2^(1/2)*dtheta^2*l_CW*cos(delta2 + theta)*sin(delta2 + pi/4)*(4*Mw + Mwca + 2*Mwma))/2 + (2^(1/2)*dtheta^2*l_CW*cos(delta4 + theta)*sin(delta4 + pi/4)*(4*Mw + Mwca + 2*Mwma))/2 ;
 (l_CW*s_w*(4*Mw + Mwca + 2*Mwma)*(cos(delta2)*(dtheta*((l_CW*cos(delta2) - l_CW*sin(delta2))/s_w - 1) + (dyc*cos(delta2 + theta))/s_w - (dxc*sin(delta2 + theta))/s_w)^2 - cos(delta1)*(dtheta*((l_CW*cos(delta1) + l_CW*sin(delta1))/s_w - 1) + (dyc*cos(delta1 + theta))/s_w - (dxc*sin(delta1 + theta))/s_w)^2 + cos(delta3)*(dtheta*((l_CW*cos(delta3) + l_CW*sin(delta3))/s_w + 1) - (dyc*cos(delta3 + theta))/s_w + (dxc*sin(delta3 + theta))/s_w)^2 - cos(delta4)*(dtheta*((l_CW*cos(delta4) - l_CW*sin(delta4))/s_w + 1) - (dyc*cos(delta4 + theta))/s_w + (dxc*sin(delta4 + theta))/s_w)^2 + sin(delta1)*(dtheta*((l_CW*cos(delta1) + l_CW*sin(delta1))/s_w - 1) + (dyc*cos(delta1 + theta))/s_w - (dxc*sin(delta1 + theta))/s_w)^2 + sin(delta2)*(dtheta*((l_CW*cos(delta2) - l_CW*sin(delta2))/s_w - 1) + (dyc*cos(delta2 + theta))/s_w - (dxc*sin(delta2 + theta))/s_w)^2 - sin(delta3)*(dtheta*((l_CW*cos(delta3) + l_CW*sin(delta3))/s_w + 1) - (dyc*cos(delta3 + theta))/s_w + (dxc*sin(delta3 + theta))/s_w)^2 - sin(delta4)*(dtheta*((l_CW*cos(delta4) - l_CW*sin(delta4))/s_w + 1) - (dyc*cos(delta4 + theta))/s_w + (dxc*sin(delta4 + theta))/s_w)^2 - 2*dtheta*cos(delta1)*(dtheta*((l_CW*cos(delta1) + l_CW*sin(delta1))/s_w - 1) + (dyc*cos(delta1 + theta))/s_w - (dxc*sin(delta1 + theta))/s_w) + 2*dtheta*cos(delta2)*(dtheta*((l_CW*cos(delta2) - l_CW*sin(delta2))/s_w - 1) + (dyc*cos(delta2 + theta))/s_w - (dxc*sin(delta2 + theta))/s_w) - 2*dtheta*cos(delta3)*(dtheta*((l_CW*cos(delta3) + l_CW*sin(delta3))/s_w + 1) - (dyc*cos(delta3 + theta))/s_w + (dxc*sin(delta3 + theta))/s_w) + 2*dtheta*cos(delta4)*(dtheta*((l_CW*cos(delta4) - l_CW*sin(delta4))/s_w + 1) - (dyc*cos(delta4 + theta))/s_w + (dxc*sin(delta4 + theta))/s_w) + 2*dtheta*sin(delta1)*(dtheta*((l_CW*cos(delta1) + l_CW*sin(delta1))/s_w - 1) + (dyc*cos(delta1 + theta))/s_w - (dxc*sin(delta1 + theta))/s_w) + 2*dtheta*sin(delta2)*(dtheta*((l_CW*cos(delta2) - l_CW*sin(delta2))/s_w - 1) + (dyc*cos(delta2 + theta))/s_w - (dxc*sin(delta2 + theta))/s_w) + 2*dtheta*sin(delta3)*(dtheta*((l_CW*cos(delta3) + l_CW*sin(delta3))/s_w + 1) - (dyc*cos(delta3 + theta))/s_w + (dxc*sin(delta3 + theta))/s_w) + 2*dtheta*sin(delta4)*(dtheta*((l_CW*cos(delta4) - l_CW*sin(delta4))/s_w + 1) - (dyc*cos(delta4 + theta))/s_w + (dxc*sin(delta4 + theta))/s_w)))/2 - dxc*((cos(delta1 + theta)*(ddelta1 + dtheta)*(Iwca + Iwma + 2*Iwz + ((l_CW*cos(delta1) + l_CW*sin(delta1))/s_w - 1)*(Iwca + Iwma + 2*Iwz + (Mw*d_w^2)/2 + 2*Mw*s_w^2 + (Mwca*s_w^2)/4 + Mwma*s_w^2) + (Mw*d_w^2)/2 + 2*Mw*s_w^2 + (Mwca*s_w^2)/4 + Mwma*s_w^2 - 2*Mw*l_CW*s_w*cos(delta1) - (Mwca*l_CW*s_w*cos(delta1))/2 - Mwma*l_CW*s_w*cos(delta1) - 2*Mw*l_CW*s_w*sin(delta1) - (Mwca*l_CW*s_w*sin(delta1))/2 - Mwma*l_CW*s_w*sin(delta1)))/s_w + (cos(delta2 + theta)*(ddelta2 + dtheta)*(Iwca + Iwma + 2*Iwz + ((l_CW*cos(delta2) - l_CW*sin(delta2))/s_w - 1)*(Iwca + Iwma + 2*Iwz + (Mw*d_w^2)/2 + 2*Mw*s_w^2 + (Mwca*s_w^2)/4 + Mwma*s_w^2) + (Mw*d_w^2)/2 + 2*Mw*s_w^2 + (Mwca*s_w^2)/4 + Mwma*s_w^2 - 2*Mw*l_CW*s_w*cos(delta2) - (Mwca*l_CW*s_w*cos(delta2))/2 - Mwma*l_CW*s_w*cos(delta2) + 2*Mw*l_CW*s_w*sin(delta2) + (Mwca*l_CW*s_w*sin(delta2))/2 + Mwma*l_CW*s_w*sin(delta2)))/s_w + (cos(delta3 + theta)*(ddelta3 + dtheta)*(Iwca + Iwma + 2*Iwz - ((l_CW*cos(delta3) + l_CW*sin(delta3))/s_w + 1)*(Iwca + Iwma + 2*Iwz + (Mw*d_w^2)/2 + 2*Mw*s_w^2 + (Mwca*s_w^2)/4 + Mwma*s_w^2) + (Mw*d_w^2)/2 + 2*Mw*s_w^2 + (Mwca*s_w^2)/4 + Mwma*s_w^2 + 2*Mw*l_CW*s_w*cos(delta3) + (Mwca*l_CW*s_w*cos(delta3))/2 + Mwma*l_CW*s_w*cos(delta3) + 2*Mw*l_CW*s_w*sin(delta3) + (Mwca*l_CW*s_w*sin(delta3))/2 + Mwma*l_CW*s_w*sin(delta3)))/s_w + (cos(delta4 + theta)*(ddelta4 + dtheta)*(Iwca + Iwma + 2*Iwz - ((l_CW*cos(delta4) - l_CW*sin(delta4))/s_w + 1)*(Iwca + Iwma + 2*Iwz + (Mw*d_w^2)/2 + 2*Mw*s_w^2 + (Mwca*s_w^2)/4 + Mwma*s_w^2) + (Mw*d_w^2)/2 + 2*Mw*s_w^2 + (Mwca*s_w^2)/4 + Mwma*s_w^2 + 2*Mw*l_CW*s_w*cos(delta4) + (Mwca*l_CW*s_w*cos(delta4))/2 + Mwma*l_CW*s_w*cos(delta4) - 2*Mw*l_CW*s_w*sin(delta4) - (Mwca*l_CW*s_w*sin(delta4))/2 - Mwma*l_CW*s_w*sin(delta4)))/s_w - (Iwp*l_CW*(sin(delta1 + theta)*(ddelta1 + dtheta) - (d_w*cos(delta1 + theta)*(ddelta1 + dtheta))/(2*s_w))*(d_w*cos(delta1) + 2*s_w*cos(delta1) + d_w*sin(delta1) - 2*s_w*sin(delta1)))/(2*r_w^2*s_w) + (Iwp*l_CW*(sin(delta1 + theta)*(ddelta1 + dtheta) + (d_w*cos(delta1 + theta)*(ddelta1 + dtheta))/(2*s_w))*(d_w*cos(delta1) - 2*s_w*cos(delta1) + d_w*sin(delta1) + 2*s_w*sin(delta1)))/(2*r_w^2*s_w) + (Iwp*l_CW*(sin(delta2 + theta)*(ddelta2 + dtheta) - (d_w*cos(delta2 + theta)*(ddelta2 + dtheta))/(2*s_w))*(2*s_w*cos(delta2) - d_w*cos(delta2) + d_w*sin(delta2) + 2*s_w*sin(delta2)))/(2*r_w^2*s_w) + (Iwp*l_CW*(sin(delta2 + theta)*(ddelta2 + dtheta) + (d_w*cos(delta2 + theta)*(ddelta2 + dtheta))/(2*s_w))*(d_w*cos(delta2) + 2*s_w*cos(delta2) - d_w*sin(delta2) + 2*s_w*sin(delta2)))/(2*r_w^2*s_w) + (Iwp*l_CW*(sin(delta3 + theta)*(ddelta3 + dtheta) - (d_w*cos(delta3 + theta)*(ddelta3 + dtheta))/(2*s_w))*(d_w*cos(delta3) + 2*s_w*cos(delta3) + d_w*sin(delta3) - 2*s_w*sin(delta3)))/(2*r_w^2*s_w) - (Iwp*l_CW*(sin(delta3 + theta)*(ddelta3 + dtheta) + (d_w*cos(delta3 + theta)*(ddelta3 + dtheta))/(2*s_w))*(d_w*cos(delta3) - 2*s_w*cos(delta3) + d_w*sin(delta3) + 2*s_w*sin(delta3)))/(2*r_w^2*s_w) - (Iwp*l_CW*(sin(delta4 + theta)*(ddelta4 + dtheta) - (d_w*cos(delta4 + theta)*(ddelta4 + dtheta))/(2*s_w))*(2*s_w*cos(delta4) - d_w*cos(delta4) + d_w*sin(delta4) + 2*s_w*sin(delta4)))/(2*r_w^2*s_w) - (Iwp*l_CW*(sin(delta4 + theta)*(ddelta4 + dtheta) + (d_w*cos(delta4 + theta)*(ddelta4 + dtheta))/(2*s_w))*(d_w*cos(delta4) + 2*s_w*cos(delta4) - d_w*sin(delta4) + 2*s_w*sin(delta4)))/(2*r_w^2*s_w)) - dyc*((sin(delta1 + theta)*(ddelta1 + dtheta)*(Iwca + Iwma + 2*Iwz + ((l_CW*cos(delta1) + l_CW*sin(delta1))/s_w - 1)*(Iwca + Iwma + 2*Iwz + (Mw*d_w^2)/2 + 2*Mw*s_w^2 + (Mwca*s_w^2)/4 + Mwma*s_w^2) + (Mw*d_w^2)/2 + 2*Mw*s_w^2 + (Mwca*s_w^2)/4 + Mwma*s_w^2 - 2*Mw*l_CW*s_w*cos(delta1) - (Mwca*l_CW*s_w*cos(delta1))/2 - Mwma*l_CW*s_w*cos(delta1) - 2*Mw*l_CW*s_w*sin(delta1) - (Mwca*l_CW*s_w*sin(delta1))/2 - Mwma*l_CW*s_w*sin(delta1)))/s_w + (sin(delta2 + theta)*(ddelta2 + dtheta)*(Iwca + Iwma + 2*Iwz + ((l_CW*cos(delta2) - l_CW*sin(delta2))/s_w - 1)*(Iwca + Iwma + 2*Iwz + (Mw*d_w^2)/2 + 2*Mw*s_w^2 + (Mwca*s_w^2)/4 + Mwma*s_w^2) + (Mw*d_w^2)/2 + 2*Mw*s_w^2 + (Mwca*s_w^2)/4 + Mwma*s_w^2 - 2*Mw*l_CW*s_w*cos(delta2) - (Mwca*l_CW*s_w*cos(delta2))/2 - Mwma*l_CW*s_w*cos(delta2) + 2*Mw*l_CW*s_w*sin(delta2) + (Mwca*l_CW*s_w*sin(delta2))/2 + Mwma*l_CW*s_w*sin(delta2)))/s_w + (sin(delta3 + theta)*(ddelta3 + dtheta)*(Iwca + Iwma + 2*Iwz - ((l_CW*cos(delta3) + l_CW*sin(delta3))/s_w + 1)*(Iwca + Iwma + 2*Iwz + (Mw*d_w^2)/2 + 2*Mw*s_w^2 + (Mwca*s_w^2)/4 + Mwma*s_w^2) + (Mw*d_w^2)/2 + 2*Mw*s_w^2 + (Mwca*s_w^2)/4 + Mwma*s_w^2 + 2*Mw*l_CW*s_w*cos(delta3) + (Mwca*l_CW*s_w*cos(delta3))/2 + Mwma*l_CW*s_w*cos(delta3) + 2*Mw*l_CW*s_w*sin(delta3) + (Mwca*l_CW*s_w*sin(delta3))/2 + Mwma*l_CW*s_w*sin(delta3)))/s_w + (sin(delta4 + theta)*(ddelta4 + dtheta)*(Iwca + Iwma + 2*Iwz - ((l_CW*cos(delta4) - l_CW*sin(delta4))/s_w + 1)*(Iwca + Iwma + 2*Iwz + (Mw*d_w^2)/2 + 2*Mw*s_w^2 + (Mwca*s_w^2)/4 + Mwma*s_w^2) + (Mw*d_w^2)/2 + 2*Mw*s_w^2 + (Mwca*s_w^2)/4 + Mwma*s_w^2 + 2*Mw*l_CW*s_w*cos(delta4) + (Mwca*l_CW*s_w*cos(delta4))/2 + Mwma*l_CW*s_w*cos(delta4) - 2*Mw*l_CW*s_w*sin(delta4) - (Mwca*l_CW*s_w*sin(delta4))/2 - Mwma*l_CW*s_w*sin(delta4)))/s_w - (Iwp*l_CW*(cos(delta1 + theta)*(ddelta1 + dtheta) - (d_w*sin(delta1 + theta)*(ddelta1 + dtheta))/(2*s_w))*(d_w*cos(delta1) - 2*s_w*cos(delta1) + d_w*sin(delta1) + 2*s_w*sin(delta1)))/(2*r_w^2*s_w) + (Iwp*l_CW*(cos(delta1 + theta)*(ddelta1 + dtheta) + (d_w*sin(delta1 + theta)*(ddelta1 + dtheta))/(2*s_w))*(d_w*cos(delta1) + 2*s_w*cos(delta1) + d_w*sin(delta1) - 2*s_w*sin(delta1)))/(2*r_w^2*s_w) - (Iwp*l_CW*(cos(delta2 + theta)*(ddelta2 + dtheta) - (d_w*sin(delta2 + theta)*(ddelta2 + dtheta))/(2*s_w))*(d_w*cos(delta2) + 2*s_w*cos(delta2) - d_w*sin(delta2) + 2*s_w*sin(delta2)))/(2*r_w^2*s_w) - (Iwp*l_CW*(cos(delta2 + theta)*(ddelta2 + dtheta) + (d_w*sin(delta2 + theta)*(ddelta2 + dtheta))/(2*s_w))*(2*s_w*cos(delta2) - d_w*cos(delta2) + d_w*sin(delta2) + 2*s_w*sin(delta2)))/(2*r_w^2*s_w) + (Iwp*l_CW*(cos(delta3 + theta)*(ddelta3 + dtheta) - (d_w*sin(delta3 + theta)*(ddelta3 + dtheta))/(2*s_w))*(d_w*cos(delta3) - 2*s_w*cos(delta3) + d_w*sin(delta3) + 2*s_w*sin(delta3)))/(2*r_w^2*s_w) - (Iwp*l_CW*(cos(delta3 + theta)*(ddelta3 + dtheta) + (d_w*sin(delta3 + theta)*(ddelta3 + dtheta))/(2*s_w))*(d_w*cos(delta3) + 2*s_w*cos(delta3) + d_w*sin(delta3) - 2*s_w*sin(delta3)))/(2*r_w^2*s_w) + (Iwp*l_CW*(cos(delta4 + theta)*(ddelta4 + dtheta) - (d_w*sin(delta4 + theta)*(ddelta4 + dtheta))/(2*s_w))*(d_w*cos(delta4) + 2*s_w*cos(delta4) - d_w*sin(delta4) + 2*s_w*sin(delta4)))/(2*r_w^2*s_w) + (Iwp*l_CW*(cos(delta4 + theta)*(ddelta4 + dtheta) + (d_w*sin(delta4 + theta)*(ddelta4 + dtheta))/(2*s_w))*(2*s_w*cos(delta4) - d_w*cos(delta4) + d_w*sin(delta4) + 2*s_w*sin(delta4)))/(2*r_w^2*s_w)) - dtheta*(((ddelta1*l_CW*sin(delta1) - ddelta1*l_CW*cos(delta1))*(Iwca + Iwma + 2*Iwz + ((l_CW*cos(delta1) + l_CW*sin(delta1))/s_w - 1)*(Iwca + Iwma + 2*Iwz + (Mw*d_w^2)/2 + 2*Mw*s_w^2 + (Mwca*s_w^2)/4 + Mwma*s_w^2) + (Mw*d_w^2)/2 + 2*Mw*s_w^2 + (Mwca*s_w^2)/4 + Mwma*s_w^2 - 2*Mw*l_CW*s_w*cos(delta1) - (Mwca*l_CW*s_w*cos(delta1))/2 - Mwma*l_CW*s_w*cos(delta1) - 2*Mw*l_CW*s_w*sin(delta1) - (Mwca*l_CW*s_w*sin(delta1))/2 - Mwma*l_CW*s_w*sin(delta1)))/s_w + ((ddelta2*l_CW*sin(delta2) + ddelta2*l_CW*cos(delta2))*(Iwca + Iwma + 2*Iwz + ((l_CW*cos(delta2) - l_CW*sin(delta2))/s_w - 1)*(Iwca + Iwma + 2*Iwz + (Mw*d_w^2)/2 + 2*Mw*s_w^2 + (Mwca*s_w^2)/4 + Mwma*s_w^2) + (Mw*d_w^2)/2 + 2*Mw*s_w^2 + (Mwca*s_w^2)/4 + Mwma*s_w^2 - 2*Mw*l_CW*s_w*cos(delta2) - (Mwca*l_CW*s_w*cos(delta2))/2 - Mwma*l_CW*s_w*cos(delta2) + 2*Mw*l_CW*s_w*sin(delta2) + (Mwca*l_CW*s_w*sin(delta2))/2 + Mwma*l_CW*s_w*sin(delta2)))/s_w - ((ddelta3*l_CW*sin(delta3) - ddelta3*l_CW*cos(delta3))*(Iwca + Iwma + 2*Iwz - ((l_CW*cos(delta3) + l_CW*sin(delta3))/s_w + 1)*(Iwca + Iwma + 2*Iwz + (Mw*d_w^2)/2 + 2*Mw*s_w^2 + (Mwca*s_w^2)/4 + Mwma*s_w^2) + (Mw*d_w^2)/2 + 2*Mw*s_w^2 + (Mwca*s_w^2)/4 + Mwma*s_w^2 + 2*Mw*l_CW*s_w*cos(delta3) + (Mwca*l_CW*s_w*cos(delta3))/2 + Mwma*l_CW*s_w*cos(delta3) + 2*Mw*l_CW*s_w*sin(delta3) + (Mwca*l_CW*s_w*sin(delta3))/2 + Mwma*l_CW*s_w*sin(delta3)))/s_w - ((ddelta4*l_CW*sin(delta4) + ddelta4*l_CW*cos(delta4))*(Iwca + Iwma + 2*Iwz - ((l_CW*cos(delta4) - l_CW*sin(delta4))/s_w + 1)*(Iwca + Iwma + 2*Iwz + (Mw*d_w^2)/2 + 2*Mw*s_w^2 + (Mwca*s_w^2)/4 + Mwma*s_w^2) + (Mw*d_w^2)/2 + 2*Mw*s_w^2 + (Mwca*s_w^2)/4 + Mwma*s_w^2 + 2*Mw*l_CW*s_w*cos(delta4) + (Mwca*l_CW*s_w*cos(delta4))/2 + Mwma*l_CW*s_w*cos(delta4) - 2*Mw*l_CW*s_w*sin(delta4) - (Mwca*l_CW*s_w*sin(delta4))/2 - Mwma*l_CW*s_w*sin(delta4)))/s_w + (Iwp*l_CW^2*(d_w*ddelta1*sin(delta1) + 2*ddelta1*s_w*sin(delta1) - d_w*ddelta1*cos(delta1) + 2*ddelta1*s_w*cos(delta1))*(d_w*cos(delta1) + 2*s_w*cos(delta1) + d_w*sin(delta1) - 2*s_w*sin(delta1)))/(4*r_w^2*s_w^2) - (Iwp*l_CW^2*(2*ddelta1*s_w*sin(delta1) - d_w*ddelta1*sin(delta1) + d_w*ddelta1*cos(delta1) + 2*ddelta1*s_w*cos(delta1))*(d_w*cos(delta1) - 2*s_w*cos(delta1) + d_w*sin(delta1) + 2*s_w*sin(delta1)))/(4*r_w^2*s_w^2) - (Iwp*l_CW^2*(d_w*ddelta2*sin(delta2) - 2*ddelta2*s_w*sin(delta2) + d_w*ddelta2*cos(delta2) + 2*ddelta2*s_w*cos(delta2))*(2*s_w*cos(delta2) - d_w*cos(delta2) + d_w*sin(delta2) + 2*s_w*sin(delta2)))/(4*r_w^2*s_w^2) + (Iwp*l_CW^2*(d_w*ddelta2*sin(delta2) + 2*ddelta2*s_w*sin(delta2) + d_w*ddelta2*cos(delta2) - 2*ddelta2*s_w*cos(delta2))*(d_w*cos(delta2) + 2*s_w*cos(delta2) - d_w*sin(delta2) + 2*s_w*sin(delta2)))/(4*r_w^2*s_w^2) + (Iwp*l_CW^2*(d_w*ddelta3*sin(delta3) + 2*ddelta3*s_w*sin(delta3) - d_w*ddelta3*cos(delta3) + 2*ddelta3*s_w*cos(delta3))*(d_w*cos(delta3) + 2*s_w*cos(delta3) + d_w*sin(delta3) - 2*s_w*sin(delta3)))/(4*r_w^2*s_w^2) - (Iwp*l_CW^2*(2*ddelta3*s_w*sin(delta3) - d_w*ddelta3*sin(delta3) + d_w*ddelta3*cos(delta3) + 2*ddelta3*s_w*cos(delta3))*(d_w*cos(delta3) - 2*s_w*cos(delta3) + d_w*sin(delta3) + 2*s_w*sin(delta3)))/(4*r_w^2*s_w^2) - (Iwp*l_CW^2*(d_w*ddelta4*sin(delta4) - 2*ddelta4*s_w*sin(delta4) + d_w*ddelta4*cos(delta4) + 2*ddelta4*s_w*cos(delta4))*(2*s_w*cos(delta4) - d_w*cos(delta4) + d_w*sin(delta4) + 2*s_w*sin(delta4)))/(4*r_w^2*s_w^2) + (Iwp*l_CW^2*(d_w*ddelta4*sin(delta4) + 2*ddelta4*s_w*sin(delta4) + d_w*ddelta4*cos(delta4) - 2*ddelta4*s_w*cos(delta4))*(d_w*cos(delta4) + 2*s_w*cos(delta4) - d_w*sin(delta4) + 2*s_w*sin(delta4)))/(4*r_w^2*s_w^2)) + (2^(1/2)*dtheta^2*l_CW*s_w*cos(delta1 + pi/4)*((l_CW*cos(delta1) + l_CW*sin(delta1))/s_w - 1)*(4*Mw + Mwca + 2*Mwma))/2 + (2^(1/2)*dtheta^2*l_CW*s_w*cos(delta3 + pi/4)*((l_CW*cos(delta3) + l_CW*sin(delta3))/s_w + 1)*(4*Mw + Mwca + 2*Mwma))/2 - (2^(1/2)*dtheta^2*l_CW*s_w*sin(delta2 + pi/4)*((l_CW*cos(delta2) - l_CW*sin(delta2))/s_w - 1)*(4*Mw + Mwca + 2*Mwma))/2 - (2^(1/2)*dtheta^2*l_CW*s_w*sin(delta4 + pi/4)*((l_CW*cos(delta4) - l_CW*sin(delta4))/s_w + 1)*(4*Mw + Mwca + 2*Mwma))/2 ;
 ];


end

== matlab function ROPOD_dynamic_model_sim_Wheel_Input/ROPOD/GtS_matrix ==
  data: ropod_dynmodel_pv input; GtS output; qin input
function GtS   = GtS_matrix( ropod_dynmodel_pv, qin)
%ROPOD_JACOBIAN Summary of this function goes here
%   Detailed explanation goes here


r_w     = ropod_dynmodel_pv(1);
s_w     = ropod_dynmodel_pv(2);
d_w     = ropod_dynmodel_pv(3);
l_CW    = ropod_dynmodel_pv(4);

Mr = ropod_dynmodel_pv(5);
Ir = ropod_dynmodel_pv(6);
Mwma = ropod_dynmodel_pv(7);
Iwma = ropod_dynmodel_pv(8);
Mwca = ropod_dynmodel_pv(9);
Iwca = ropod_dynmodel_pv(10);
Mw   = ropod_dynmodel_pv(11);
Iwz  = ropod_dynmodel_pv(12);
Iwp  = ropod_dynmodel_pv(13);


% Map state vector to the corresponfing variables
xc      = qin(1);
yc      = qin(2);
theta   = qin(3);
delta   = qin(4:7);
varphi  = qin(8:15);

delta1 = delta(1);
delta2 = delta(2);
delta3 = delta(3);
delta4 = delta(4);

GtS = [
    [                                   (cos(delta1 + theta) + (d_w*sin(delta1 + theta))/(2*s_w))/r_w,                                  (cos(delta1 + theta) - (d_w*sin(delta1 + theta))/(2*s_w))/r_w,                                  (cos(delta2 + theta) + (d_w*sin(delta2 + theta))/(2*s_w))/r_w,                                  (cos(delta2 + theta) - (d_w*sin(delta2 + theta))/(2*s_w))/r_w,                                  (cos(delta3 + theta) + (d_w*sin(delta3 + theta))/(2*s_w))/r_w,                                   (cos(delta3 + theta) - (d_w*sin(delta3 + theta))/(2*s_w))/r_w,                                   (cos(delta4 + theta) + (d_w*sin(delta4 + theta))/(2*s_w))/r_w,                                   (cos(delta4 + theta) - (d_w*sin(delta4 + theta))/(2*s_w))/r_w]
    [                                   (sin(delta1 + theta) - (d_w*cos(delta1 + theta))/(2*s_w))/r_w,                                  (sin(delta1 + theta) + (d_w*cos(delta1 + theta))/(2*s_w))/r_w,                                  (sin(delta2 + theta) - (d_w*cos(delta2 + theta))/(2*s_w))/r_w,                                  (sin(delta2 + theta) + (d_w*cos(delta2 + theta))/(2*s_w))/r_w,                                  (sin(delta3 + theta) - (d_w*cos(delta3 + theta))/(2*s_w))/r_w,                                   (sin(delta3 + theta) + (d_w*cos(delta3 + theta))/(2*s_w))/r_w,                                   (sin(delta4 + theta) - (d_w*cos(delta4 + theta))/(2*s_w))/r_w,                                   (sin(delta4 + theta) + (d_w*cos(delta4 + theta))/(2*s_w))/r_w]
    [ -(l_CW*(d_w*cos(delta1) + 2*s_w*cos(delta1) + d_w*sin(delta1) - 2*s_w*sin(delta1)))/(2*r_w*s_w), (l_CW*(d_w*cos(delta1) - 2*s_w*cos(delta1) + d_w*sin(delta1) + 2*s_w*sin(delta1)))/(2*r_w*s_w), (l_CW*(2*s_w*cos(delta2) - d_w*cos(delta2) + d_w*sin(delta2) + 2*s_w*sin(delta2)))/(2*r_w*s_w), (l_CW*(d_w*cos(delta2) + 2*s_w*cos(delta2) - d_w*sin(delta2) + 2*s_w*sin(delta2)))/(2*r_w*s_w), (l_CW*(d_w*cos(delta3) + 2*s_w*cos(delta3) + d_w*sin(delta3) - 2*s_w*sin(delta3)))/(2*r_w*s_w), -(l_CW*(d_w*cos(delta3) - 2*s_w*cos(delta3) + d_w*sin(delta3) + 2*s_w*sin(delta3)))/(2*r_w*s_w), -(l_CW*(2*s_w*cos(delta4) - d_w*cos(delta4) + d_w*sin(delta4) + 2*s_w*sin(delta4)))/(2*r_w*s_w), -(l_CW*(d_w*cos(delta4) + 2*s_w*cos(delta4) - d_w*sin(delta4) + 2*s_w*sin(delta4)))/(2*r_w*s_w)] 
 ];


end

== matlab function ROPOD_dynamic_model_sim_Wheel_Input/Feedback Linearization/JqwT_matrix_c ==
  data: ropod_dynmodel_pv input; JqwT output; qin input
function JqwT   = JqwT_matrix( ropod_dynmodel_pv, qin)
%ROPOD_JACOBIAN Summary of this function goes here
%   Detailed explanation goes here


r_w     = ropod_dynmodel_pv(1);
s_w     = ropod_dynmodel_pv(2);
d_w     = ropod_dynmodel_pv(3);
l_CW    = ropod_dynmodel_pv(4);

Mr = ropod_dynmodel_pv(5);
Ir = ropod_dynmodel_pv(6);
Mwma = ropod_dynmodel_pv(7);
Iwma = ropod_dynmodel_pv(8);
Mwca = ropod_dynmodel_pv(9);
Iwca = ropod_dynmodel_pv(10);
Mw   = ropod_dynmodel_pv(11);
Iwz  = ropod_dynmodel_pv(12);
Iwp  = ropod_dynmodel_pv(13);


% Map state vector to the corresponfing variables
xc      = qin(1);
yc      = qin(2);
theta   = qin(3);
delta   = qin(4:7);
varphi  = qin(8:15);

delta1 = delta(1);
delta2 = delta(2);
delta3 = delta(3);
delta4 = delta(4);

JqwT = [
[ (r_w*(d_w*cos(delta1 + theta) + 2*s_w*sin(delta1 + theta)))/(8*d_w), -(r_w*(2*s_w*cos(delta1 + theta) - d_w*sin(delta1 + theta)))/(8*d_w), -(r_w*(d_w*cos(delta1) + 2*s_w*cos(delta1) - d_w*sin(delta1) + 2*s_w*sin(delta1)))/(16*d_w*l_CW)]
[ (r_w*(d_w*cos(delta1 + theta) - 2*s_w*sin(delta1 + theta)))/(8*d_w),  (r_w*(2*s_w*cos(delta1 + theta) + d_w*sin(delta1 + theta)))/(8*d_w),  (r_w*(2*s_w*cos(delta1) - d_w*cos(delta1) + d_w*sin(delta1) + 2*s_w*sin(delta1)))/(16*d_w*l_CW)]
[ (r_w*(d_w*cos(delta2 + theta) + 2*s_w*sin(delta2 + theta)))/(8*d_w), -(r_w*(2*s_w*cos(delta2 + theta) - d_w*sin(delta2 + theta)))/(8*d_w),  (r_w*(d_w*cos(delta2) - 2*s_w*cos(delta2) + d_w*sin(delta2) + 2*s_w*sin(delta2)))/(16*d_w*l_CW)]
[ (r_w*(d_w*cos(delta2 + theta) - 2*s_w*sin(delta2 + theta)))/(8*d_w),  (r_w*(2*s_w*cos(delta2 + theta) + d_w*sin(delta2 + theta)))/(8*d_w),  (r_w*(d_w*cos(delta2) + 2*s_w*cos(delta2) + d_w*sin(delta2) - 2*s_w*sin(delta2)))/(16*d_w*l_CW)]
[ (r_w*(d_w*cos(delta3 + theta) + 2*s_w*sin(delta3 + theta)))/(8*d_w), -(r_w*(2*s_w*cos(delta3 + theta) - d_w*sin(delta3 + theta)))/(8*d_w),  (r_w*(d_w*cos(delta3) + 2*s_w*cos(delta3) - d_w*sin(delta3) + 2*s_w*sin(delta3)))/(16*d_w*l_CW)]
[ (r_w*(d_w*cos(delta3 + theta) - 2*s_w*sin(delta3 + theta)))/(8*d_w),  (r_w*(2*s_w*cos(delta3 + theta) + d_w*sin(delta3 + theta)))/(8*d_w), -(r_w*(2*s_w*cos(delta3) - d_w*cos(delta3) + d_w*sin(delta3) + 2*s_w*sin(delta3)))/(16*d_w*l_CW)]
[ (r_w*(d_w*cos(delta4 + theta) + 2*s_w*sin(delta4 + theta)))/(8*d_w), -(r_w*(2*s_w*cos(delta4 + theta) - d_w*sin(delta4 + theta)))/(8*d_w), -(r_w*(d_w*cos(delta4) - 2*s_w*cos(delta4) + d_w*sin(delta4) + 2*s_w*sin(delta4)))/(16*d_w*l_CW)]
[ (r_w*(d_w*cos(delta4 + theta) - 2*s_w*sin(delta4 + theta)))/(8*d_w),  (r_w*(2*s_w*cos(delta4 + theta) + d_w*sin(delta4 + theta)))/(8*d_w), -(r_w*(d_w*cos(delta4) + 2*s_w*cos(delta4) + d_w*sin(delta4) - 2*s_w*sin(delta4)))/(16*d_w*l_CW)]
];


end
